simulink model "CTC"  (R2022b)
settings: Solver=VariableStepAuto  StartTime=0.0  StopTime=30  RelTol=1e-3
model workspace (MATLAB code in the model file):
  other statements: smiData.RigidTransform(98).translation = [0.0 0.0 0.0];; smiData.RigidTransform(98).angle = 0.0;; smiData.RigidTransform(98).axis = [0.0 0.0 0.0];; smiData.RigidTransform(98).ID = '';; smiData.RigidTransform(1).translation = [0 19.999999999999989 175];  % mm; smiData.RigidTransform(1).angle = 2.0943951023931953;  % rad; smiData.RigidTransform(1).axis = [0.57735026918962584 -0.57735026918962584 0.57735026918962584];; smiData.RigidTransform(1).ID = 'B[UpperLeg_2:Upper_Leg-1:-:UpperLeg_2:Joint_1-1]';; smiData.RigidTransform(2).translation = [-10.000000000089699 -1.8161827597396041e-10 -1.8518164779379731e-10];  % mm; smiData.RigidTransform(2).angle = 2.0943951023931953;  % rad; smiData.RigidTransform(2).axis = [0.57735026918962618 0.57735026918962562 0.5773502691896254];; smiData.RigidTransform(2).ID = 'F[UpperLeg_2:Upper_Leg-1:-:UpperLeg_2:Joint_1-1]'; ... (+537)
undefined symbols (not defined in the file): DiscIntNeverNeededParam, smiData, X, Y, Z
libraries: sm_lib x246, nesl_utility x13
(part 6 of 6)

== system CTC/Subsystem/LowerLeg_Assembly2_6_RIGID/Lower_Leg_1_RIGID ==
  ReferenceFrame : sm_lib/Frames and Transforms/Reference Frame
  Solid : sm_lib/Body Elements/File Solid  ExtGeomFileName=C:\Users\FPTSHOP\Desktop\IUD LAB\Delta Robot\Model_2\3.lower_leg\Lower_Leg.SLDPRT  UnitType=FromFile  ExtGeomFileUnits=m  StepReaderType=HEX  ExportConvexHullGeometry=off  InertiaType=Custom  Mass=smiData.Solid(4).mass  MassUnits=kg  CenterOfMass=smiData.Solid(4).CoM  CenterOfMassUnits=mm  MomentsOfInertia=smiData.Solid(4).MoI  MomentsOfInertiaUnits=kg*mm^2  ProductsOfInertia=smiData.Solid(4).PoI  ProductsOfInertiaUnits=kg*mm^2  BasedOnType=DensityFromFile  Density=1000  DensityUnits=kg/m^3  DoExposeReferenceFrame=on  SerializedFrames=<Frames/>  GraphicType=FromGeometry  MarkerShape=Sphere  MarkerSize=10  GraphicVisPropType=SimpleVisualProperties  GraphicDiffuseColor=smiData.Solid(4).color  GraphicSpecularColor=[0.5 0.5 0.5 1.0]  GraphicAmbientColor=[0.15 0.15 0.15 1.0]  GraphicEmissiveColor=[0.0 0.0 0.0 1.0]  GraphicShininess=75  GraphicOpacity=smiData.Solid(4).opacity
  F : PMIOPort  Side=Left
  connections:
  Solid/RConn1 -- ReferenceFrame/RConn1 -- F/RConn1

== system CTC/Subsystem/UpperLeg_2_3/Joint_1_1_RIGID ==
  ReferenceFrame : sm_lib/Frames and Transforms/Reference Frame
  Solid : sm_lib/Body Elements/File Solid  ExtGeomFileName=C:\Users\FPTSHOP\Desktop\IUD LAB\Delta Robot\Model_2\3.lower_leg\Joint_1.SLDPRT  UnitType=FromFile  ExtGeomFileUnits=m  StepReaderType=HEX  ExportConvexHullGeometry=off  InertiaType=Custom  Mass=smiData.Solid(2).mass  MassUnits=kg  CenterOfMass=smiData.Solid(2).CoM  CenterOfMassUnits=mm  MomentsOfInertia=smiData.Solid(2).MoI  MomentsOfInertiaUnits=kg*mm^2  ProductsOfInertia=smiData.Solid(2).PoI  ProductsOfInertiaUnits=kg*mm^2  BasedOnType=DensityFromFile  Density=1000  DensityUnits=kg/m^3  DoExposeReferenceFrame=on  SerializedFrames=<Frames/>  GraphicType=FromGeometry  MarkerShape=Sphere  MarkerSize=10  GraphicVisPropType=SimpleVisualProperties  GraphicDiffuseColor=smiData.Solid(2).color  GraphicSpecularColor=[0.5 0.5 0.5 1.0]  GraphicAmbientColor=[0.15 0.15 0.15 1.0]  GraphicEmissiveColor=[0.0 0.0 0.0 1.0]  GraphicShininess=75  GraphicOpacity=smiData.Solid(2).opacity
  Transform : sm_lib/Frames and Transforms/Rigid Transform  TranslationMethod=Cartesian  TranslationStandardOffset=0  TranslationLengthUnit=mm  TranslationStandardAxis=+Z  TranslationCartesianOffset=smiData.RigidTransform(2).translation  TranslationROffset=0  TranslationROffsetUnits=m  TranslationZOffset=0  TranslationZOffsetUnits=m  TranslationThetaOffset=0  TranslationThetaOffsetUnits=deg  RotationMethod=ArbitraryAxis  RotationAngleUnits=rad  RotationStandardAxis=+Z  RotationAngle=smiData.RigidTransform(2).angle  RotationArbitraryAxis=smiData.RigidTransform(2).axis  FollAlignAxisA=+X  BaseAlignAxisA=+Y  FollAlignAxisB=+Y  BaseAlignAxisB=+Z  RotationSequenceAxes=FollowerAxes  RotationSequence=XYX  RotationSequenceAngles=[0 0 0]  RotationSequenceAnglesUnits=deg  RotationMatrix=[1 0 0; 0 1 0; 0 0 1]  Quaternion=[1 0 0 0]
  Transform1 : sm_lib/Frames and Transforms/Rigid Transform  TranslationMethod=Cartesian  TranslationStandardOffset=0  TranslationLengthUnit=mm  TranslationStandardAxis=+Z  TranslationCartesianOffset=smiData.RigidTransform(11).translation  TranslationROffset=0  TranslationROffsetUnits=m  TranslationZOffset=0  TranslationZOffsetUnits=m  TranslationThetaOffset=0  TranslationThetaOffsetUnits=deg  RotationMethod=ArbitraryAxis  RotationAngleUnits=rad  RotationStandardAxis=+Z  RotationAngle=smiData.RigidTransform(11).angle  RotationArbitraryAxis=smiData.RigidTransform(11).axis  FollAlignAxisA=+X  BaseAlignAxisA=+Y  FollAlignAxisB=+Y  BaseAlignAxisB=+Z  RotationSequenceAxes=FollowerAxes  RotationSequence=XYX  RotationSequenceAngles=[0 0 0]  RotationSequenceAnglesUnits=deg  RotationMatrix=[1 0 0; 0 1 0; 0 0 1]  Quaternion=[1 0 0 0]
  Transform2 : sm_lib/Frames and Transforms/Rigid Transform  TranslationMethod=Cartesian  TranslationStandardOffset=0  TranslationLengthUnit=mm  TranslationStandardAxis=+Z  TranslationCartesianOffset=smiData.RigidTransform(21).translation  TranslationROffset=0  TranslationROffsetUnits=m  TranslationZOffset=0  TranslationZOffsetUnits=m  TranslationThetaOffset=0  TranslationThetaOffsetUnits=deg  RotationMethod=ArbitraryAxis  RotationAngleUnits=rad  RotationStandardAxis=+Z  RotationAngle=smiData.RigidTransform(21).angle  RotationArbitraryAxis=smiData.RigidTransform(21).axis  FollAlignAxisA=+X  BaseAlignAxisA=+Y  FollAlignAxisB=+Y  BaseAlignAxisB=+Z  RotationSequenceAxes=FollowerAxes  RotationSequence=XYX  RotationSequenceAngles=[0 0 0]  RotationSequenceAnglesUnits=deg  RotationMatrix=[1 0 0; 0 1 0; 0 0 1]  Quaternion=[1 0 0 0]
  Transform3 : sm_lib/Frames and Transforms/Rigid Transform  TranslationMethod=Cartesian  TranslationStandardOffset=0  TranslationLengthUnit=mm  TranslationStandardAxis=+Z  TranslationCartesianOffset=smiData.RigidTransform(25).translation  TranslationROffset=0  TranslationROffsetUnits=m  TranslationZOffset=0  TranslationZOffsetUnits=m  TranslationThetaOffset=0  TranslationThetaOffsetUnits=deg  RotationMethod=ArbitraryAxis  RotationAngleUnits=rad  RotationStandardAxis=+Z  RotationAngle=smiData.RigidTransform(25).angle  RotationArbitraryAxis=smiData.RigidTransform(25).axis  FollAlignAxisA=+X  BaseAlignAxisA=+Y  FollAlignAxisB=+Y  BaseAlignAxisB=+Z  RotationSequenceAxes=FollowerAxes  RotationSequence=XYX  RotationSequenceAngles=[0 0 0]  RotationSequenceAnglesUnits=deg  RotationMatrix=[1 0 0; 0 1 0; 0 0 1]  Quaternion=[1 0 0 0]
  Transform4 : sm_lib/Frames and Transforms/Rigid Transform  TranslationMethod=Cartesian  TranslationStandardOffset=0  TranslationLengthUnit=mm  TranslationStandardAxis=+Z  TranslationCartesianOffset=smiData.RigidTransform(67).translation  TranslationROffset=0  TranslationROffsetUnits=m  TranslationZOffset=0  TranslationZOffsetUnits=m  TranslationThetaOffset=0  TranslationThetaOffsetUnits=deg  RotationMethod=ArbitraryAxis  RotationAngleUnits=rad  RotationStandardAxis=+Z  RotationAngle=smiData.RigidTransform(67).angle  RotationArbitraryAxis=smiData.RigidTransform(67).axis  FollAlignAxisA=+X  BaseAlignAxisA=+Y  FollAlignAxisB=+Y  BaseAlignAxisB=+Z  RotationSequenceAxes=FollowerAxes  RotationSequence=XYX  RotationSequenceAngles=[0 0 0]  RotationSequenceAnglesUnits=deg  RotationMatrix=[1 0 0; 0 1 0; 0 0 1]  Quaternion=[1 0 0 0]
  F1 : PMIOPort  Side=Left
  F2 : PMIOPort  Port=2  Side=Left
  F3 : PMIOPort  Port=3  Side=Left
  F4 : PMIOPort  Port=4  Side=Left
  F : PMIOPort  Port=5  Side=Left
  connections:
  Solid/RConn1 -- ReferenceFrame/RConn1 -- Transform/LConn1 -- Transform1/LConn1 -- Transform3/LConn1 -- Transform4/LConn1 -- Transform2/LConn1
  Transform/RConn1 -- F/RConn1
  Transform1/RConn1 -- F1/RConn1
  Transform2/RConn1 -- F2/RConn1
  Transform3/RConn1 -- F3/RConn1
  Transform4/RConn1 -- F4/RConn1

== system CTC/Subsystem/UpperLeg_2_3/Upper_Leg_1_RIGID ==
  ReferenceFrame : sm_lib/Frames and Transforms/Reference Frame
  Solid : sm_lib/Body Elements/File Solid  ExtGeomFileName=C:\Users\FPTSHOP\Desktop\IUD LAB\Delta Robot\Model_2\2.upper_leg\Upper_Leg.SLDPRT  UnitType=FromFile  ExtGeomFileUnits=m  StepReaderType=HEX  ExportConvexHullGeometry=off  InertiaType=Custom  Mass=smiData.Solid(1).mass  MassUnits=kg  CenterOfMass=smiData.Solid(1).CoM  CenterOfMassUnits=mm  MomentsOfInertia=smiData.Solid(1).MoI  MomentsOfInertiaUnits=kg*mm^2  ProductsOfInertia=smiData.Solid(1).PoI  ProductsOfInertiaUnits=kg*mm^2  BasedOnType=DensityFromFile  Density=1000  DensityUnits=kg/m^3  DoExposeReferenceFrame=on  SerializedFrames=<Frames/>  GraphicType=FromGeometry  MarkerShape=Sphere  MarkerSize=10  GraphicVisPropType=SimpleVisualProperties  GraphicDiffuseColor=smiData.Solid(1).color  GraphicSpecularColor=[0.5 0.5 0.5 1.0]  GraphicAmbientColor=[0.15 0.15 0.15 1.0]  GraphicEmissiveColor=[0.0 0.0 0.0 1.0]  GraphicShininess=75  GraphicOpacity=smiData.Solid(1).opacity
  Transform : sm_lib/Frames and Transforms/Rigid Transform  TranslationMethod=Cartesian  TranslationStandardOffset=0  TranslationLengthUnit=mm  TranslationStandardAxis=+Z  TranslationCartesianOffset=smiData.RigidTransform(1).translation  TranslationROffset=0  TranslationROffsetUnits=m  TranslationZOffset=0  TranslationZOffsetUnits=m  TranslationThetaOffset=0  TranslationThetaOffsetUnits=deg  RotationMethod=ArbitraryAxis  RotationAngleUnits=rad  RotationStandardAxis=+Z  RotationAngle=smiData.RigidTransform(1).angle  RotationArbitraryAxis=smiData.RigidTransform(1).axis  FollAlignAxisA=+X  BaseAlignAxisA=+Y  FollAlignAxisB=+Y  BaseAlignAxisB=+Z  RotationSequenceAxes=FollowerAxes  RotationSequence=XYX  RotationSequenceAngles=[0 0 0]  RotationSequenceAnglesUnits=deg  RotationMatrix=[1 0 0; 0 1 0; 0 0 1]  Quaternion=[1 0 0 0]
  Transform1 : sm_lib/Frames and Transforms/Rigid Transform  TranslationMethod=Cartesian  TranslationStandardOffset=0  TranslationLengthUnit=mm  TranslationStandardAxis=+Z  TranslationCartesianOffset=smiData.RigidTransform(42).translation  TranslationROffset=0  TranslationROffsetUnits=m  TranslationZOffset=0  TranslationZOffsetUnits=m  TranslationThetaOffset=0  TranslationThetaOffsetUnits=deg  RotationMethod=ArbitraryAxis  RotationAngleUnits=rad  RotationStandardAxis=+Z  RotationAngle=smiData.RigidTransform(42).angle  RotationArbitraryAxis=smiData.RigidTransform(42).axis  FollAlignAxisA=+X  BaseAlignAxisA=+Y  FollAlignAxisB=+Y  BaseAlignAxisB=+Z  RotationSequenceAxes=FollowerAxes  RotationSequence=XYX  RotationSequenceAngles=[0 0 0]  RotationSequenceAnglesUnits=deg  RotationMatrix=[1 0 0; 0 1 0; 0 0 1]  Quaternion=[1 0 0 0]
  F2 : PMIOPort  Side=Left
  F1 : PMIOPort  Port=2  Side=Left
  F : PMIOPort  Port=3  Side=Right
  connections:
  Solid/RConn1 -- ReferenceFrame/RConn1 -- Transform/LConn1 -- Transform1/LConn1 -- F2/RConn1
  Transform/RConn1 -- F/RConn1
  Transform1/RConn1 -- F1/RConn1

== system CTC/Subsystem/UpperLeg_2_4/Joint_1_1_RIGID ==
  ReferenceFrame : sm_lib/Frames and Transforms/Reference Frame
  Solid : sm_lib/Body Elements/File Solid  ExtGeomFileName=C:\Users\FPTSHOP\Desktop\IUD LAB\Delta Robot\Model_2\3.lower_leg\Joint_1.SLDPRT  UnitType=FromFile  ExtGeomFileUnits=m  StepReaderType=HEX  ExportConvexHullGeometry=off  InertiaType=Custom  Mass=smiData.Solid(2).mass  MassUnits=kg  CenterOfMass=smiData.Solid(2).CoM  CenterOfMassUnits=mm  MomentsOfInertia=smiData.Solid(2).MoI  MomentsOfInertiaUnits=kg*mm^2  ProductsOfInertia=smiData.Solid(2).PoI  ProductsOfInertiaUnits=kg*mm^2  BasedOnType=DensityFromFile  Density=1000  DensityUnits=kg/m^3  DoExposeReferenceFrame=on  SerializedFrames=<Frames/>  GraphicType=FromGeometry  MarkerShape=Sphere  MarkerSize=10  GraphicVisPropType=SimpleVisualProperties  GraphicDiffuseColor=smiData.Solid(2).color  GraphicSpecularColor=[0.5 0.5 0.5 1.0]  GraphicAmbientColor=[0.15 0.15 0.15 1.0]  GraphicEmissiveColor=[0.0 0.0 0.0 1.0]  GraphicShininess=75  GraphicOpacity=smiData.Solid(2).opacity
  Transform : sm_lib/Frames and Transforms/Rigid Transform  TranslationMethod=Cartesian  TranslationStandardOffset=0  TranslationLengthUnit=mm  TranslationStandardAxis=+Z  TranslationCartesianOffset=smiData.RigidTransform(2).translation  TranslationROffset=0  TranslationROffsetUnits=m  TranslationZOffset=0  TranslationZOffsetUnits=m  TranslationThetaOffset=0  TranslationThetaOffsetUnits=deg  RotationMethod=ArbitraryAxis  RotationAngleUnits=rad  RotationStandardAxis=+Z  RotationAngle=smiData.RigidTransform(2).angle  RotationArbitraryAxis=smiData.RigidTransform(2).axis  FollAlignAxisA=+X  BaseAlignAxisA=+Y  FollAlignAxisB=+Y  BaseAlignAxisB=+Z  RotationSequenceAxes=FollowerAxes  RotationSequence=XYX  RotationSequenceAngles=[0 0 0]  RotationSequenceAnglesUnits=deg  RotationMatrix=[1 0 0; 0 1 0; 0 0 1]  Quaternion=[1 0 0 0]
  Transform1 : sm_lib/Frames and Transforms/Rigid Transform  TranslationMethod=Cartesian  TranslationStandardOffset=0  TranslationLengthUnit=mm  TranslationStandardAxis=+Z  TranslationCartesianOffset=smiData.RigidTransform(29).translation  TranslationROffset=0  TranslationROffsetUnits=m  TranslationZOffset=0  TranslationZOffsetUnits=m  TranslationThetaOffset=0  TranslationThetaOffsetUnits=deg  RotationMethod=ArbitraryAxis  RotationAngleUnits=rad  RotationStandardAxis=+Z  RotationAngle=smiData.RigidTransform(29).angle  RotationArbitraryAxis=smiData.RigidTransform(29).axis  FollAlignAxisA=+X  BaseAlignAxisA=+Y  FollAlignAxisB=+Y  BaseAlignAxisB=+Z  RotationSequenceAxes=FollowerAxes  RotationSequence=XYX  RotationSequenceAngles=[0 0 0]  RotationSequenceAnglesUnits=deg  RotationMatrix=[1 0 0; 0 1 0; 0 0 1]  Quaternion=[1 0 0 0]
  Transform2 : sm_lib/Frames and Transforms/Rigid Transform  TranslationMethod=Cartesian  TranslationStandardOffset=0  TranslationLengthUnit=mm  TranslationStandardAxis=+Z  TranslationCartesianOffset=smiData.RigidTransform(33).translation  TranslationROffset=0  TranslationROffsetUnits=m  TranslationZOffset=0  TranslationZOffsetUnits=m  TranslationThetaOffset=0  TranslationThetaOffsetUnits=deg  RotationMethod=ArbitraryAxis  RotationAngleUnits=rad  RotationStandardAxis=+Z  RotationAngle=smiData.RigidTransform(33).angle  RotationArbitraryAxis=smiData.RigidTransform(33).axis  FollAlignAxisA=+X  BaseAlignAxisA=+Y  FollAlignAxisB=+Y  BaseAlignAxisB=+Z  RotationSequenceAxes=FollowerAxes  RotationSequence=XYX  RotationSequenceAngles=[0 0 0]  RotationSequenceAnglesUnits=deg  RotationMatrix=[1 0 0; 0 1 0; 0 0 1]  Quaternion=[1 0 0 0]
  Transform3 : sm_lib/Frames and Transforms/Rigid Transform  TranslationMethod=Cartesian  TranslationStandardOffset=0  TranslationLengthUnit=mm  TranslationStandardAxis=+Z  TranslationCartesianOffset=smiData.RigidTransform(47).translation  TranslationROffset=0  TranslationROffsetUnits=m  TranslationZOffset=0  TranslationZOffsetUnits=m  TranslationThetaOffset=0  TranslationThetaOffsetUnits=deg  RotationMethod=ArbitraryAxis  RotationAngleUnits=rad  RotationStandardAxis=+Z  RotationAngle=smiData.RigidTransform(47).angle  RotationArbitraryAxis=smiData.RigidTransform(47).axis  FollAlignAxisA=+X  BaseAlignAxisA=+Y  FollAlignAxisB=+Y  BaseAlignAxisB=+Z  RotationSequenceAxes=FollowerAxes  RotationSequence=XYX  RotationSequenceAngles=[0 0 0]  RotationSequenceAnglesUnits=deg  RotationMatrix=[1 0 0; 0 1 0; 0 0 1]  Quaternion=[1 0 0 0]
  Transform4 : sm_lib/Frames and Transforms/Rigid Transform  TranslationMethod=Cartesian  TranslationStandardOffset=0  TranslationLengthUnit=mm  TranslationStandardAxis=+Z  TranslationCartesianOffset=smiData.RigidTransform(51).translation  TranslationROffset=0  TranslationROffsetUnits=m  TranslationZOffset=0  TranslationZOffsetUnits=m  TranslationThetaOffset=0  TranslationThetaOffsetUnits=deg  RotationMethod=ArbitraryAxis  RotationAngleUnits=rad  RotationStandardAxis=+Z  RotationAngle=smiData.RigidTransform(51).angle  RotationArbitraryAxis=smiData.RigidTransform(51).axis  FollAlignAxisA=+X  BaseAlignAxisA=+Y  FollAlignAxisB=+Y  BaseAlignAxisB=+Z  RotationSequenceAxes=FollowerAxes  RotationSequence=XYX  RotationSequenceAngles=[0 0 0]  RotationSequenceAnglesUnits=deg  RotationMatrix=[1 0 0; 0 1 0; 0 0 1]  Quaternion=[1 0 0 0]
  F1 : PMIOPort  Side=Left
  F2 : PMIOPort  Port=2  Side=Left
  F3 : PMIOPort  Port=3  Side=Left
  F4 : PMIOPort  Port=4  Side=Left
  F : PMIOPort  Port=5  Side=Left
  connections:
  Solid/RConn1 -- ReferenceFrame/RConn1 -- Transform/LConn1 -- Transform1/LConn1 -- Transform3/LConn1 -- Transform4/LConn1 -- Transform2/LConn1
  Transform/RConn1 -- F/RConn1
  Transform1/RConn1 -- F1/RConn1
  Transform2/RConn1 -- F2/RConn1
  Transform3/RConn1 -- F3/RConn1
  Transform4/RConn1 -- F4/RConn1

== system CTC/Subsystem/UpperLeg_2_4/Upper_Leg_1_RIGID ==
  ReferenceFrame : sm_lib/Frames and Transforms/Reference Frame
  Solid : sm_lib/Body Elements/File Solid  ExtGeomFileName=C:\Users\FPTSHOP\Desktop\IUD LAB\Delta Robot\Model_2\2.upper_leg\Upper_Leg.SLDPRT  UnitType=FromFile  ExtGeomFileUnits=m  StepReaderType=HEX  ExportConvexHullGeometry=off  InertiaType=Custom  Mass=smiData.Solid(1).mass  MassUnits=kg  CenterOfMass=smiData.Solid(1).CoM  CenterOfMassUnits=mm  MomentsOfInertia=smiData.Solid(1).MoI  MomentsOfInertiaUnits=kg*mm^2  ProductsOfInertia=smiData.Solid(1).PoI  ProductsOfInertiaUnits=kg*mm^2  BasedOnType=DensityFromFile  Density=1000  DensityUnits=kg/m^3  DoExposeReferenceFrame=on  SerializedFrames=<Frames/>  GraphicType=FromGeometry  MarkerShape=Sphere  MarkerSize=10  GraphicVisPropType=SimpleVisualProperties  GraphicDiffuseColor=smiData.Solid(1).color  GraphicSpecularColor=[0.5 0.5 0.5 1.0]  GraphicAmbientColor=[0.15 0.15 0.15 1.0]  GraphicEmissiveColor=[0.0 0.0 0.0 1.0]  GraphicShininess=75  GraphicOpacity=smiData.Solid(1).opacity
  Transform : sm_lib/Frames and Transforms/Rigid Transform  TranslationMethod=Cartesian  TranslationStandardOffset=0  TranslationLengthUnit=mm  TranslationStandardAxis=+Z  TranslationCartesianOffset=smiData.RigidTransform(1).translation  TranslationROffset=0  TranslationROffsetUnits=m  TranslationZOffset=0  TranslationZOffsetUnits=m  TranslationThetaOffset=0  TranslationThetaOffsetUnits=deg  RotationMethod=ArbitraryAxis  RotationAngleUnits=rad  RotationStandardAxis=+Z  RotationAngle=smiData.RigidTransform(1).angle  RotationArbitraryAxis=smiData.RigidTransform(1).axis  FollAlignAxisA=+X  BaseAlignAxisA=+Y  FollAlignAxisB=+Y  BaseAlignAxisB=+Z  RotationSequenceAxes=FollowerAxes  RotationSequence=XYX  RotationSequenceAngles=[0 0 0]  RotationSequenceAnglesUnits=deg  RotationMatrix=[1 0 0; 0 1 0; 0 0 1]  Quaternion=[1 0 0 0]
  Transform1 : sm_lib/Frames and Transforms/Rigid Transform  TranslationMethod=Cartesian  TranslationStandardOffset=0  TranslationLengthUnit=mm  TranslationStandardAxis=+Z  TranslationCartesianOffset=smiData.RigidTransform(40).translation  TranslationROffset=0  TranslationROffsetUnits=m  TranslationZOffset=0  TranslationZOffsetUnits=m  TranslationThetaOffset=0  TranslationThetaOffsetUnits=deg  RotationMethod=ArbitraryAxis  RotationAngleUnits=rad  RotationStandardAxis=+Z  RotationAngle=smiData.RigidTransform(40).angle  RotationArbitraryAxis=smiData.RigidTransform(40).axis  FollAlignAxisA=+X  BaseAlignAxisA=+Y  FollAlignAxisB=+Y  BaseAlignAxisB=+Z  RotationSequenceAxes=FollowerAxes  RotationSequence=XYX  RotationSequenceAngles=[0 0 0]  RotationSequenceAnglesUnits=deg  RotationMatrix=[1 0 0; 0 1 0; 0 0 1]  Quaternion=[1 0 0 0]
  F2 : PMIOPort  Side=Left
  F1 : PMIOPort  Port=2  Side=Left
  F : PMIOPort  Port=3  Side=Right
  connections:
  Solid/RConn1 -- ReferenceFrame/RConn1 -- Transform/LConn1 -- Transform1/LConn1 -- F2/RConn1
  Transform/RConn1 -- F/RConn1
  Transform1/RConn1 -- F1/RConn1

== system CTC/Subsystem/UpperLeg_2_5/Joint_1_1_RIGID ==
  ReferenceFrame : sm_lib/Frames and Transforms/Reference Frame
  Solid : sm_lib/Body Elements/File Solid  ExtGeomFileName=C:\Users\FPTSHOP\Desktop\IUD LAB\Delta Robot\Model_2\3.lower_leg\Joint_1.SLDPRT  UnitType=FromFile  ExtGeomFileUnits=m  StepReaderType=HEX  ExportConvexHullGeometry=off  InertiaType=Custom  Mass=smiData.Solid(2).mass  MassUnits=kg  CenterOfMass=smiData.Solid(2).CoM  CenterOfMassUnits=mm  MomentsOfInertia=smiData.Solid(2).MoI  MomentsOfInertiaUnits=kg*mm^2  ProductsOfInertia=smiData.Solid(2).PoI  ProductsOfInertiaUnits=kg*mm^2  BasedOnType=DensityFromFile  Density=1000  DensityUnits=kg/m^3  DoExposeReferenceFrame=on  SerializedFrames=<Frames/>  GraphicType=FromGeometry  MarkerShape=Sphere  MarkerSize=10  GraphicVisPropType=SimpleVisualProperties  GraphicDiffuseColor=smiData.Solid(2).color  GraphicSpecularColor=[0.5 0.5 0.5 1.0]  GraphicAmbientColor=[0.15 0.15 0.15 1.0]  GraphicEmissiveColor=[0.0 0.0 0.0 1.0]  GraphicShininess=75  GraphicOpacity=smiData.Solid(2).opacity
  Transform : sm_lib/Frames and Transforms/Rigid Transform  TranslationMethod=Cartesian  TranslationStandardOffset=0  TranslationLengthUnit=mm  TranslationStandardAxis=+Z  TranslationCartesianOffset=smiData.RigidTransform(2).translation  TranslationROffset=0  TranslationROffsetUnits=m  TranslationZOffset=0  TranslationZOffsetUnits=m  TranslationThetaOffset=0  TranslationThetaOffsetUnits=deg  RotationMethod=ArbitraryAxis  RotationAngleUnits=rad  RotationStandardAxis=+Z  RotationAngle=smiData.RigidTransform(2).angle  RotationArbitraryAxis=smiData.RigidTransform(2).axis  FollAlignAxisA=+X  BaseAlignAxisA=+Y  FollAlignAxisB=+Y  BaseAlignAxisB=+Z  RotationSequenceAxes=FollowerAxes  RotationSequence=XYX  RotationSequenceAngles=[0 0 0]  RotationSequenceAnglesUnits=deg  RotationMatrix=[1 0 0; 0 1 0; 0 0 1]  Quaternion=[1 0 0 0]
  Transform1 : sm_lib/Frames and Transforms/Rigid Transform  TranslationMethod=Cartesian  TranslationStandardOffset=0  TranslationLengthUnit=mm  TranslationStandardAxis=+Z  TranslationCartesianOffset=smiData.RigidTransform(13).translation  TranslationROffset=0  TranslationROffsetUnits=m  TranslationZOffset=0  TranslationZOffsetUnits=m  TranslationThetaOffset=0  TranslationThetaOffsetUnits=deg  RotationMethod=ArbitraryAxis  RotationAngleUnits=rad  RotationStandardAxis=+Z  RotationAngle=smiData.RigidTransform(13).angle  RotationArbitraryAxis=smiData.RigidTransform(13).axis  FollAlignAxisA=+X  BaseAlignAxisA=+Y  FollAlignAxisB=+Y  BaseAlignAxisB=+Z  RotationSequenceAxes=FollowerAxes  RotationSequence=XYX  RotationSequenceAngles=[0 0 0]  RotationSequenceAnglesUnits=deg  RotationMatrix=[1 0 0; 0 1 0; 0 0 1]  Quaternion=[1 0 0 0]
  Transform2 : sm_lib/Frames and Transforms/Rigid Transform  TranslationMethod=Cartesian  TranslationStandardOffset=0  TranslationLengthUnit=mm  TranslationStandardAxis=+Z  TranslationCartesianOffset=smiData.RigidTransform(15).translation  TranslationROffset=0  TranslationROffsetUnits=m  TranslationZOffset=0  TranslationZOffsetUnits=m  TranslationThetaOffset=0  TranslationThetaOffsetUnits=deg  RotationMethod=ArbitraryAxis  RotationAngleUnits=rad  RotationStandardAxis=+Z  RotationAngle=smiData.RigidTransform(15).angle  RotationArbitraryAxis=smiData.RigidTransform(15).axis  FollAlignAxisA=+X  BaseAlignAxisA=+Y  FollAlignAxisB=+Y  BaseAlignAxisB=+Z  RotationSequenceAxes=FollowerAxes  RotationSequence=XYX  RotationSequenceAngles=[0 0 0]  RotationSequenceAnglesUnits=deg  RotationMatrix=[1 0 0; 0 1 0; 0 0 1]  Quaternion=[1 0 0 0]
  Transform3 : sm_lib/Frames and Transforms/Rigid Transform  TranslationMethod=Cartesian  TranslationStandardOffset=0  TranslationLengthUnit=mm  TranslationStandardAxis=+Z  TranslationCartesianOffset=smiData.RigidTransform(43).translation  TranslationROffset=0  TranslationROffsetUnits=m  TranslationZOffset=0  TranslationZOffsetUnits=m  TranslationThetaOffset=0  TranslationThetaOffsetUnits=deg  RotationMethod=ArbitraryAxis  RotationAngleUnits=rad  RotationStandardAxis=+Z  RotationAngle=smiData.RigidTransform(43).angle  RotationArbitraryAxis=smiData.RigidTransform(43).axis  FollAlignAxisA=+X  BaseAlignAxisA=+Y  FollAlignAxisB=+Y  BaseAlignAxisB=+Z  RotationSequenceAxes=FollowerAxes  RotationSequence=XYX  RotationSequenceAngles=[0 0 0]  RotationSequenceAnglesUnits=deg  RotationMatrix=[1 0 0; 0 1 0; 0 0 1]  Quaternion=[1 0 0 0]
  Transform4 : sm_lib/Frames and Transforms/Rigid Transform  TranslationMethod=Cartesian  TranslationStandardOffset=0  TranslationLengthUnit=mm  TranslationStandardAxis=+Z  TranslationCartesianOffset=smiData.RigidTransform(45).translation  TranslationROffset=0  TranslationROffsetUnits=m  TranslationZOffset=0  TranslationZOffsetUnits=m  TranslationThetaOffset=0  TranslationThetaOffsetUnits=deg  RotationMethod=ArbitraryAxis  RotationAngleUnits=rad  RotationStandardAxis=+Z  RotationAngle=smiData.RigidTransform(45).angle  RotationArbitraryAxis=smiData.RigidTransform(45).axis  FollAlignAxisA=+X  BaseAlignAxisA=+Y  FollAlignAxisB=+Y  BaseAlignAxisB=+Z  RotationSequenceAxes=FollowerAxes  RotationSequence=XYX  RotationSequenceAngles=[0 0 0]  RotationSequenceAnglesUnits=deg  RotationMatrix=[1 0 0; 0 1 0; 0 0 1]  Quaternion=[1 0 0 0]
  F1 : PMIOPort  Side=Left
  F2 : PMIOPort  Port=2  Side=Left
  F3 : PMIOPort  Port=3  Side=Left
  F4 : PMIOPort  Port=4  Side=Left
  F : PMIOPort  Port=5  Side=Left
  connections:
  Solid/RConn1 -- ReferenceFrame/RConn1 -- Transform/LConn1 -- Transform1/LConn1 -- Transform3/LConn1 -- Transform4/LConn1 -- Transform2/LConn1
  Transform/RConn1 -- F/RConn1
  Transform1/RConn1 -- F1/RConn1
  Transform2/RConn1 -- F2/RConn1
  Transform3/RConn1 -- F3/RConn1
  Transform4/RConn1 -- F4/RConn1

== system CTC/Subsystem/UpperLeg_2_5/Upper_Leg_1_RIGID ==
  ReferenceFrame : sm_lib/Frames and Transforms/Reference Frame
  Solid : sm_lib/Body Elements/File Solid  ExtGeomFileName=C:\Users\FPTSHOP\Desktop\IUD LAB\Delta Robot\Model_2\2.upper_leg\Upper_Leg.SLDPRT  UnitType=FromFile  ExtGeomFileUnits=m  StepReaderType=HEX  ExportConvexHullGeometry=off  InertiaType=Custom  Mass=smiData.Solid(1).mass  MassUnits=kg  CenterOfMass=smiData.Solid(1).CoM  CenterOfMassUnits=mm  MomentsOfInertia=smiData.Solid(1).MoI  MomentsOfInertiaUnits=kg*mm^2  ProductsOfInertia=smiData.Solid(1).PoI  ProductsOfInertiaUnits=kg*mm^2  BasedOnType=DensityFromFile  Density=1000  DensityUnits=kg/m^3  DoExposeReferenceFrame=on  SerializedFrames=<Frames/>  GraphicType=FromGeometry  MarkerShape=Sphere  MarkerSize=10  GraphicVisPropType=SimpleVisualProperties  GraphicDiffuseColor=smiData.Solid(1).color  GraphicSpecularColor=[0.5 0.5 0.5 1.0]  GraphicAmbientColor=[0.15 0.15 0.15 1.0]  GraphicEmissiveColor=[0.0 0.0 0.0 1.0]  GraphicShininess=75  GraphicOpacity=smiData.Solid(1).opacity
  Transform : sm_lib/Frames and Transforms/Rigid Transform  TranslationMethod=Cartesian  TranslationStandardOffset=0  TranslationLengthUnit=mm  TranslationStandardAxis=+Z  TranslationCartesianOffset=smiData.RigidTransform(1).translation  TranslationROffset=0  TranslationROffsetUnits=m  TranslationZOffset=0  TranslationZOffsetUnits=m  TranslationThetaOffset=0  TranslationThetaOffsetUnits=deg  RotationMethod=ArbitraryAxis  RotationAngleUnits=rad  RotationStandardAxis=+Z  RotationAngle=smiData.RigidTransform(1).angle  RotationArbitraryAxis=smiData.RigidTransform(1).axis  FollAlignAxisA=+X  BaseAlignAxisA=+Y  FollAlignAxisB=+Y  BaseAlignAxisB=+Z  RotationSequenceAxes=FollowerAxes  RotationSequence=XYX  RotationSequenceAngles=[0 0 0]  RotationSequenceAnglesUnits=deg  RotationMatrix=[1 0 0; 0 1 0; 0 0 1]  Quaternion=[1 0 0 0]
  Transform1 : sm_lib/Frames and Transforms/Rigid Transform  TranslationMethod=Cartesian  TranslationStandardOffset=0  TranslationLengthUnit=mm  TranslationStandardAxis=+Z  TranslationCartesianOffset=smiData.RigidTransform(18).translation  TranslationROffset=0  TranslationROffsetUnits=m  TranslationZOffset=0  TranslationZOffsetUnits=m  TranslationThetaOffset=0  TranslationThetaOffsetUnits=deg  RotationMethod=ArbitraryAxis  RotationAngleUnits=rad  RotationStandardAxis=+Z  RotationAngle=smiData.RigidTransform(18).angle  RotationArbitraryAxis=smiData.RigidTransform(18).axis  FollAlignAxisA=+X  BaseAlignAxisA=+Y  FollAlignAxisB=+Y  BaseAlignAxisB=+Z  RotationSequenceAxes=FollowerAxes  RotationSequence=XYX  RotationSequenceAngles=[0 0 0]  RotationSequenceAnglesUnits=deg  RotationMatrix=[1 0 0; 0 1 0; 0 0 1]  Quaternion=[1 0 0 0]
  F2 : PMIOPort  Side=Left
  F1 : PMIOPort  Port=2  Side=Left
  F : PMIOPort  Port=3  Side=Right
  connections:
  Solid/RConn1 -- ReferenceFrame/RConn1 -- Transform/LConn1 -- Transform1/LConn1 -- F2/RConn1
  Transform/RConn1 -- F/RConn1
  Transform1/RConn1 -- F1/RConn1

== matlab function CTC/Subsystem11/MATLAB Function3 ==
  settings: updateMethod=DISCRETE
  data: u input; cl input; y output
function y = fcn(u, cl)
    persistent mark;  % Declare 'mark' as a persistent variable

    if isempty(mark)
        mark = 0;  % Default initialization if 'mark' is not yet defined
    end

    if (cl == 0)
        mark = u;  % Store the first data when cl is 0
        y = u;     % Output the first data
    elseif (cl >= 0.01 && cl <= 0.5)
        y = mark;  % Output the stored data when cl is between 0.01 and 0.05
    else
        y = 0;     % Set a default value for other cases if needed
    end
end

== matlab function CTC/MATLAB Function3 ==
  data: out output; theta1_dd input; theta2_dd input; theta3_dd input
function out = fcn(theta1_dd, theta2_dd, theta3_dd)
out = [theta1_dd; theta2_dd; theta3_dd];

== matlab function CTC/MATLAB Function5 ==
  data: M output
function M = massMatrix()

m2 = 0.017070467811714975 + (5.04 + 0.79*2 + 1.81*2)*10^-3;
rf = 175*10^-3;
I1 = 1094992.78 * 10^-9;

M = diag([I1 + m2*rf^2,I1 + m2*rf^2,I1 + m2*rf^2]);

== matlab function CTC/Subsystem2/MATLAB Function4 ==
  data: theta1 input; lambda1 output; theta2 input; theta3 input; x input; y input; z input; x_dd input; y_dd input; z_dd input; lambda2 output; lambda3 output
function [lambda1, lambda2, lambda3] = LagrangeMultipliers(theta1, theta2, theta3, x, y, z, x_dd, y_dd, z_dd)

phi1 = pi/3;
phi2 = pi;
phi3 = -pi/3;
e = 73.76*10^-3;
f = 163.68*10^-3;
re = 372.04*10^-3;
rf = 175*10^-3;
mp = 102.96*10^-3;
m2 = 0.017070467811714975 + (5.04 + 0.79*2 + 1.81*2)*10^-3;
g = 9.81;

x = x * 10^-3;
y = y * 10^-3;
z = z * 10^-3;

R = [(mp + 3*m2)*x_dd; (mp + 3*m2)*y_dd; (mp + 3*m2)*(z_dd + g)];
L = [2*(x + e*cos(phi1) - f*cos(phi1) - rf*cos(phi1)*cos(theta1)), 2*(x + e*cos(phi2) - f*cos(phi2) - rf*cos(phi2)*cos(theta2)), 2*(x + e*cos(phi3) - f*cos(phi3) - rf*cos(phi3)*cos(theta3));
     2*(y + e*sin(phi1) - f*sin(phi1) - rf*sin(phi1)*cos(theta1)), 2*(y + e*sin(phi2) - f*sin(phi2) - rf*sin(phi2)*cos(theta2)), 2*(y + e*sin(phi3) - f*sin(phi3) - rf*sin(phi3)*cos(theta3));
     2*(z - rf*sin(theta1)), 2*(z - rf*sin(theta2)), 2*(z - rf*sin(theta3))];

res = inv(L) * R;

lambda1 = res(1);
lambda2 = res(2);
lambda3 = res(3);
end

== matlab function CTC/forwardDynamics/MATLAB Function ==
  data: torque1 input; torque output; torque2 input; torque3 input
function torque = fcn(torque1, torque2, torque3)

torque = [torque1; torque2; torque3]

== matlab function CTC/Subsystem2/MATLAB Function6 ==
  data: x input; G output; y input; z input; theta1 input; theta2 input; theta3 input; lambda1 input; lambda2 input; lambda3 input
function G = GMatrix(x, y, z, theta1, theta2, theta3, lambda1, lambda2, lambda3)

I1 = 1094992.78 * 10^-9;
m1 = 0.14169795977416536;
m2 = 0.017070467811714975 + (5.04 + 0.79*2 + 1.81*2)*10^-3;
e = 73.76*10^-3;
f = 163.68*10^-3;
re = 372.04*10^-3;
rf = 175*10^-3;
l1c = 67.023520991164446*10^-3;
phi1 = pi/3;
phi2 = pi;
phi3 = -pi/3;
g = 9.81;

x = x * 10^-3;
y = y * 10^-3;
z = z * 10^-3;

g1 = +(m1*l1c + m2*rf)*g*cos(theta1) - 2*rf*lambda1*((x*cos(phi1) + y*sin(phi1) + e - f)*sin(theta1) - z*cos(theta1));
g2 = +(m1*l1c + m2*rf)*g*cos(theta2) - 2*rf*lambda2*((x*cos(phi2) + y*sin(phi2) + e - f)*sin(theta2) - z*cos(theta2));
g3 = +(m1*l1c + m2*rf)*g*cos(theta3) - 2*rf*lambda3*((x*cos(phi3) + y*sin(phi3) + e - f)*sin(theta3) - z*cos(theta3));

G = [g1; g2; g3];

== matlab function CTC/forwardDynamics/MATLAB Function3 ==
  data: q1_dd output; torque input; M input; G input; q2_dd output; q3_dd output
function [q1_dd, q2_dd, q3_dd] = forwardDynamics(torque, M, G)



q_dd = inv(M) * (torque - G);
q1_dd = q_dd(1);
q2_dd = q_dd(2);
q3_dd = q_dd(3);

== matlab function CTC/Subsystem1/MATLAB Function3 ==
  settings: updateMethod=DISCRETE
  data: u input; cl input; y output
function y = fcn(u, cl)
    persistent mark;  % Declare 'mark' as a persistent variable

    if isempty(mark)
        mark = 0;  % Default initialization if 'mark' is not yet defined
    end

    if (cl == 0)
        mark = u;  % Store the first data when cl is 0
        y = u;     % Output the first data
    elseif (cl >= 0.01 && cl <= 0.5)
        y = mark;  % Output the stored data when cl is between 0.01 and 0.05
    else
        y = 0;     % Set a default value for other cases if needed
    end
end

== matlab function CTC/Subsystem1/MATLAB Function4 ==
  data: u1 input; y output; u2 input; cl input
function y = fcn(u1, u2, cl)

if (cl <= 0.5)
    y = u1;
else
    y = u2;
end

== matlab function CTC/Subsystem3/MATLAB Function3 ==
  settings: updateMethod=DISCRETE
  data: u input; cl input; y output
function y = fcn(u, cl)
    persistent mark;  % Declare 'mark' as a persistent variable

    if isempty(mark)
        mark = 0;  % Default initialization if 'mark' is not yet defined
    end

    if (cl == 0)
        mark = u;  % Store the first data when cl is 0
        y = u;     % Output the first data
    elseif (cl >= 0.01 && cl <= 0.5)
        y = mark;  % Output the stored data when cl is between 0.01 and 0.05
    else
        y = 0;     % Set a default value for other cases if needed
    end
end

== matlab function CTC/Subsystem3/MATLAB Function4 ==
  data: u1 input; y output; u2 input; cl input
function y = fcn(u1, u2, cl)

if (cl <= 0.5)
    y = u1;
else
    y = u2;
end

== matlab function CTC/Subsystem5/MATLAB Function3 ==
  settings: updateMethod=DISCRETE
  data: u input; cl input; y output
function y = fcn(u, cl)
    persistent mark;  % Declare 'mark' as a persistent variable

    if isempty(mark)
        mark = 0;  % Default initialization if 'mark' is not yet defined
    end

    if (cl == 0)
        mark = u;  % Store the first data when cl is 0
        y = u;     % Output the first data
    elseif (cl >= 0.01 && cl <= 0.02)
        y = mark;  % Output the stored data when cl is between 0.01 and 0.05
    else
        y = 0;     % Set a default value for other cases if needed
    end
end

== matlab function CTC/Subsystem5/MATLAB Function4 ==
  data: u1 input; y output; u2 input; cl input
function y = fcn(u1, u2, cl)

if (cl <= 0.02)
    y = u1;
else
    y = u2;
end

== matlab function CTC/Subsystem6/MATLAB Function3 ==
  settings: updateMethod=DISCRETE
  data: u input; cl input; y output
function y = fcn(u, cl)
    persistent mark;  % Declare 'mark' as a persistent variable

    if isempty(mark)
        mark = 0;  % Default initialization if 'mark' is not yet defined
    end

    if (cl == 0)
        mark = u;  % Store the first data when cl is 0
        y = u;     % Output the first data
    elseif (cl >= 0.01 && cl <= 0.02)
        y = mark;  % Output the stored data when cl is between 0.01 and 0.05
    else
        y = 0;     % Set a default value for other cases if needed
    end
end

== matlab function CTC/Subsystem6/MATLAB Function4 ==
  data: u1 input; y output; u2 input; cl input
function y = fcn(u1, u2, cl)

if (cl <= 0.02)
    y = u1;
else
    y = u2;
end

== matlab function CTC/Subsystem7/MATLAB Function4 ==
  data: u1 input; y output; u2 input; cl input
function y = fcn(u1, u2, cl)

if (cl <= 0.5)
    y = u1;
else
    y = u2;
end

== matlab function CTC/Subsystem11/MATLAB Function4 ==
  data: u1 input; y output; u2 input; cl input
function y = fcn(u1, u2, cl)

if (cl <= 0.5)
    y = u1;
else
    y = u2;
end

== matlab function CTC/Subsystem8/MATLAB Function3 ==
  settings: updateMethod=DISCRETE
  data: u input; cl input; y output
function y = fcn(u, cl)
    persistent mark;  % Declare 'mark' as a persistent variable

    if isempty(mark)
        mark = 0;  % Default initialization if 'mark' is not yet defined
    end

    if (cl == 0)
        mark = u;  % Store the first data when cl is 0
        y = u;     % Output the first data
    elseif (cl >= 0.01 && cl <= 0.02)
        y = mark;  % Output the stored data when cl is between 0.01 and 0.05
    else
        y = 0;     % Set a default value for other cases if needed
    end
end

== matlab function CTC/Subsystem8/MATLAB Function4 ==
  data: u1 input; y output; u2 input; cl input
function y = fcn(u1, u2, cl)

if (cl <= 0.02)
    y = u1;
else
    y = u2;
end

== matlab function CTC/Subsystem12/MATLAB Function3 ==
  settings: updateMethod=DISCRETE
  data: u input; cl input; y output
function y = fcn(u, cl)
    persistent mark;  % Declare 'mark' as a persistent variable

    if isempty(mark)
        mark = 0;  % Default initialization if 'mark' is not yet defined
    end

    if (cl == 0)
        mark = u;  % Store the first data when cl is 0
        y = u;     % Output the first data
    elseif (cl >= 0.01 && cl <= 0.5)
        y = mark;  % Output the stored data when cl is between 0.01 and 0.05
    else
        y = 0;     % Set a default value for other cases if needed
    end
end

== matlab function CTC/forwardDynamics/MATLAB Function5 ==
  data: M output
function M = massMatrix()

m2 = 0.017070467811714975 + (5.04 + 0.79*2 + 1.81*2)*10^-3;
rf = 175*10^-3;
I1 = 1094992.78 * 10^-9;

M = diag([I1 + m2*rf^2,I1 + m2*rf^2,I1 + m2*rf^2]);

== matlab function CTC/Subsystem12/MATLAB Function4 ==
  data: u1 input; y output; u2 input; cl input
function y = fcn(u1, u2, cl)

if (cl <= 0.5)
    y = u1;
else
    y = u2;
end

== matlab function CTC/Subsystem13/MATLAB Function3 ==
  settings: updateMethod=DISCRETE
  data: u input; cl input; y output
function y = fcn(u, cl)
    persistent mark;  % Declare 'mark' as a persistent variable

    if isempty(mark)
        mark = 0;  % Default initialization if 'mark' is not yet defined
    end

    if (cl == 0)
        mark = u;  % Store the first data when cl is 0
        y = u;     % Output the first data
    elseif (cl >= 0.01 && cl <= 0.5)
        y = mark;  % Output the stored data when cl is between 0.01 and 0.05
    else
        y = 0;     % Set a default value for other cases if needed
    end
end

== matlab function CTC/Subsystem13/MATLAB Function4 ==
  data: u1 input; y output; u2 input; cl input
function y = fcn(u1, u2, cl)

if (cl <= 0.5)
    y = u1;
else
    y = u2;
end

== matlab function CTC/Subsystem14/MATLAB Function3 ==
  settings: updateMethod=DISCRETE
  data: u input; cl input; y output
function y = fcn(u, cl)
    persistent mark;  % Declare 'mark' as a persistent variable

    if isempty(mark)
        mark = 0;  % Default initialization if 'mark' is not yet defined
    end

    if (cl == 0)
        mark = u;  % Store the first data when cl is 0
        y = u;     % Output the first data
    elseif (cl >= 0.01 && cl <= 0.5)
        y = mark;  % Output the stored data when cl is between 0.01 and 0.05
    else
        y = 0;     % Set a default value for other cases if needed
    end
end

== matlab function CTC/Subsystem14/MATLAB Function4 ==
  data: u1 input; y output; u2 input; cl input
function y = fcn(u1, u2, cl)

if (cl <= 0.5)
    y = u1;
else
    y = u2;
end

== matlab function CTC/forwardDynamics/Subsystem/MATLAB Function1 ==
  data: theta1 input; lambda1 output; theta2 input; theta3 input; x input; y input; z input; x_dd input; y_dd input; z_dd input; lambda2 output; lambda3 output
function [lambda1, lambda2, lambda3] = LagrangeMultipliers(theta1, theta2, theta3, x, y, z, x_dd, y_dd, z_dd)

phi1 = pi/3;
phi2 = pi;
phi3 = -pi/3;
e = 73.76*10^-3;
f = 163.68*10^-3;
re = 372.04*10^-3;
rf = 175*10^-3;
mp = 102.96*10^-3;
m2 = 0.017070467811714975 + (5.04 + 0.79*2 + 1.81*2)*10^-3;
g = 9.81;

x = x * 10^-3;
y = y * 10^-3;
z = z * 10^-3;

R = [(mp + 3*m2)*x_dd; (mp + 3*m2)*y_dd; (mp + 3*m2)*(z_dd + g)];
L = [2*(x + e*cos(phi1) - f*cos(phi1) - rf*cos(phi1)*cos(theta1)), 2*(x + e*cos(phi2) - f*cos(phi2) - rf*cos(phi2)*cos(theta2)), 2*(x + e*cos(phi3) - f*cos(phi3) - rf*cos(phi3)*cos(theta3));
     2*(y + e*sin(phi1) - f*sin(phi1) - rf*sin(phi1)*cos(theta1)), 2*(y + e*sin(phi2) - f*sin(phi2) - rf*sin(phi2)*cos(theta2)), 2*(y + e*sin(phi3) - f*sin(phi3) - rf*sin(phi3)*cos(theta3));
     2*(z - rf*sin(theta1)), 2*(z - rf*sin(theta2)), 2*(z - rf*sin(theta3))];

res = inv(L) * R;

lambda1 = res(1);
lambda2 = res(2);
lambda3 = res(3);
end

== matlab function CTC/forwardDynamics/Subsystem/MATLAB Function2 ==
  data: x input; G output; y input; z input; theta1 input; theta2 input; theta3 input; lambda1 input; lambda2 input; lambda3 input
function G = GMatrix(x, y, z, theta1, theta2, theta3, lambda1, lambda2, lambda3)

I1 = 1094992.78 * 10^-9;
m1 = 0.14169795977416536;
m2 = 0.017070467811714975 + (5.04 + 0.79*2 + 1.81*2)*10^-3;
e = 73.76*10^-3;
f = 163.68*10^-3;
re = 372.04*10^-3;
rf = 175*10^-3;
l1c = 67.023520991164446*10^-3;
phi1 = pi/3;
phi2 = pi;
phi3 = -pi/3;
g = 9.81;

x = x * 10^-3;
y = y * 10^-3;
z = z * 10^-3;

g1 = +(m1*l1c + m2*rf)*g*cos(theta1) - 2*rf*lambda1*((x*cos(phi1) + y*sin(phi1) + e - f)*sin(theta1) - z*cos(theta1));
g2 = +(m1*l1c + m2*rf)*g*cos(theta2) - 2*rf*lambda2*((x*cos(phi2) + y*sin(phi2) + e - f)*sin(theta2) - z*cos(theta2));
g3 = +(m1*l1c + m2*rf)*g*cos(theta3) - 2*rf*lambda3*((x*cos(phi3) + y*sin(phi3) + e - f)*sin(theta3) - z*cos(theta3));

G = [g1; g2; g3];

== matlab function CTC/Subsystem7/MATLAB Function3 ==
  settings: updateMethod=DISCRETE
  data: u input; cl input; y output
function y = fcn(u, cl)
    persistent mark;  % Declare 'mark' as a persistent variable

    if isempty(mark)
        mark = 0;  % Default initialization if 'mark' is not yet defined
    end

    if (cl == 0)
        mark = u;  % Store the first data when cl is 0
        y = u;     % Output the first data
    elseif (cl >= 0.01 && cl <= 0.5)
        y = mark;  % Output the stored data when cl is between 0.01 and 0.05
    else
        y = 0;     % Set a default value for other cases if needed
    end
end

== matlab function CTC/Subsystem9/MATLAB Function3 ==
  settings: updateMethod=DISCRETE
  data: u input; cl input; y output
function y = fcn(u, cl)
    persistent mark;  % Declare 'mark' as a persistent variable

    if isempty(mark)
        mark = 0;  % Default initialization if 'mark' is not yet defined
    end

    if (cl == 0)
        mark = u;  % Store the first data when cl is 0
        y = u;     % Output the first data
    elseif (cl >= 0.01 && cl <= 0.5)
        y = mark;  % Output the stored data when cl is between 0.01 and 0.05
    else
        y = 0;     % Set a default value for other cases if needed
    end
end

== matlab function CTC/Subsystem9/MATLAB Function4 ==
  data: u1 input; y output; u2 input; cl input
function y = fcn(u1, u2, cl)

if (cl <= 0.5)
    y = u1;
else
    y = u2;
end

== matlab function CTC/Subsystem10/MATLAB Function3 ==
  settings: updateMethod=DISCRETE
  data: u input; cl input; y output
function y = fcn(u, cl)
    persistent mark;  % Declare 'mark' as a persistent variable

    if isempty(mark)
        mark = 0;  % Default initialization if 'mark' is not yet defined
    end

    if (cl == 0)
        mark = u;  % Store the first data when cl is 0
        y = u;     % Output the first data
    elseif (cl >= 0.01 && cl <= 0.5)
        y = mark;  % Output the stored data when cl is between 0.01 and 0.05
    else
        y = 0;     % Set a default value for other cases if needed
    end
end

== matlab function CTC/Subsystem10/MATLAB Function4 ==
  data: u1 input; y output; u2 input; cl input
function y = fcn(u1, u2, cl)

if (cl <= 0.5)
    y = u1;
else
    y = u2;
end
